simulink model "IDVDSGRA_StatObs_Close"  (R2017b)
settings: Solver=ode4  StartTime=0.0  StopTime=tsim  FixedStep=baseRate  RelTol=1e-3  EnableMultiTasking=on
values from neighbouring files (symbols this model uses):
  baseRate = 0.05    [Run_Initializer.m]
  dockDist = 0.5    [Run_Initializer.m]
  drop_states_BLACK = [ 1.19; 1.45; -0.06737]    [Run_Initializer.m]
  drop_states_RED = [ 2.114; 1.46; -3.113]    [Run_Initializer.m]
  F_thrusters_BLACK = 0.25.*ones(8,1)    [Run_Initializer.m]
  F_thrusters_RED = 0.25.*ones(8,1)    [Run_Initializer.m]
  final_states_BLACK = [1; 0.5; (0/180*pi)]    [Run_Initializer.m]
  fixed_att = init_states_RED(3)    [Run_Initializer.m]
  guess = [8.968203153403679e+02,-2.543974115068790e+03,0.235869606391541,0.474952865321742,0.474987768379695,0.520000000000000,0.485664087948638,0,0,.1,.1,.1,.1,.1,.1,.1,.1,.1,.1,.1,.1,.1,.1,.1,.1,.1,.2]    [Run_Initializer.m]
  home_states_BLACK = [ xLength/2; yLength/2; 0]    [Run_Initializer.m]
  home_states_RED = [ xLength/2+0.4; yLength/2; pi]    [Run_Initializer.m]
  init_states_BLACK = [0.5; 0.5; (0/180*pi)]    [Run_Initializer.m]
  init_states_RED = [ 3; 2; 0]    [Run_Initializer.m]
  Kd_tb = 0.4    [Run_Initializer.m]
  Kd_tr = 0.4    [Run_Initializer.m]
  Kd_xb = 5    [Run_Initializer.m]
  Kd_xr = 5    [Run_Initializer.m]
  Kd_yb = 5    [Run_Initializer.m]
  Kd_yr = 5    [Run_Initializer.m]
  Kp_tb = 0.1    [Run_Initializer.m]
  Kp_tr = 0.1    [Run_Initializer.m]
  Kp_xb = 2    [Run_Initializer.m]
  Kp_xr = 2    [Run_Initializer.m]
  Kp_yb = 2    [Run_Initializer.m]
  Kp_yr = 2    [Run_Initializer.m]
  max_force = F_thrusters_RED(1)*2 * 0.95    [Run_Initializer.m]
  max_torque = 0.13*4    (= 0.52)    [Run_Initializer.m]
  moving_BLACK = [(final_states_BLACK(1)-init_states_BLACK(1))/Phase3_SubPhase2_Duration,(final_states_BLACK(2)-init_states_BLACK(2))/Phase3_SubPhase2_Duration,0]    [Run_Initializer.m]
  noise_variance_BLACK = 0    [Run_Initializer.m]
  noise_variance_RED = 0    [Run_Initializer.m]
  Phase0_End = Phase0_Duration    (= 10)    [Run_Initializer.m]
  Phase1_End = Phase0_Duration + Phase1_Duration    (= 15)    [Run_Initializer.m]
  Phase2_End = Phase0_Duration + Phase1_Duration +                                   Phase2_Duration    (= 35)    [Run_Initializer.m]
  Phase3_Duration = 85    [Run_Initializer.m]
  Phase3_End = Phase0_Duration + Phase1_Duration +                                   Phase2_Duration + Phase3_Duration    (= 120)    [Run_Initializer.m]
  Phase3_SubPhase1_End = Phase2_End + Phase3_SubPhase1_Duration    (= 40)    [Run_Initializer.m]
  Phase3_SubPhase2_Duration = 70    [Run_Initializer.m]
  Phase3_SubPhase2_End = Phase2_End + Phase3_SubPhase1_Duration +                                   Phase3_SubPhase2_Duration    (= 110)    [Run_Initializer.m]
  Phase3_SubPhase3_End = Phase2_End + Phase3_SubPhase1_Duration +                                   Phase3_SubPhase2_Duration +                                  Phase3_SubPhase3_Duration    (= 120)    [Run_Initializer.m]
  Phase3_SubPhase4_End = Phase2_End + Phase3_SubPhase1_Duration +                                   Phase3_SubPhase2_Duration +                                  Phase3_SubPhase3_Duration +                                  Phase3_SubPhase4_Duration    [Run_Initializer.m]
  Phase4_End = Phase0_Duration + Phase1_Duration +                                   Phase2_Duration + Phase3_Duration +                                   Phase4_Duration    (= 140)    [Run_Initializer.m]
  Phase5_End = Phase0_Duration + Phase1_Duration +                                   Phase2_Duration + Phase3_Duration +                                   Phase4_Duration + Phase5_Duration    (= 145)    [Run_Initializer.m]
  REDInertia = 0.2709    [Run_Initializer.m]
  REDMass = 16.9478    [Run_Initializer.m]
  serverRate = 0.1    [Run_Initializer.m]
  thruster_dist2CG_BLACK = [83.42;-52.58;55.94;-60.05;54.08;-53.92;77.06;-55.94]    [Run_Initializer.m]
  thruster_dist2CG_RED = [49.92;-78.08;70.46;-63.54;81.08;-50.42;57.44;-75.96]    [Run_Initializer.m]
  tolSGRA = [Er; Eg]    [Run_Initializer.m]
  xLength = 3.51155    [Run_Initializer.m]
  yLength = 2.41935    [Run_Initializer.m]
undefined symbols (not defined in the file or in its folder): DiscIntNeverNeededParam, platformSelection, simMode
libraries: MainLibrary x22, GPIOLibrary x20, raspberrypilib x17, embdlinuxlib x6, dspsigops x5, dspswit3 x2, simulink x1
(part 8 of 8)

== matlab function IDVDSGRA_StatObs_Close/Phase #5: Hold Home/Change BLACK Behavior/Hough Control/MATLAB Function3 ==
  data: z input; Ox output
function Ox    = C3( z )
%C3 gives the rotation matrix about the z-axis for an angle 'z'
%   z - the angle about the z-axis which you rotate
%   A - the rotation matrix

Ox = [cos(z) sin(z); -sin(z) cos(z)]*[1;0];
end

== matlab function IDVDSGRA_StatObs_Close/Phase #5: Hold Home/Change BLACK Behavior/Hough Control/MATLAB Function4 ==
  data: Oy input; e_out output; e_in input
function e_out = fcn(Oy, e_in)

a = sign(Oy'*e_in);
e_out = -a*norm(e_in);

== matlab function IDVDSGRA_StatObs_Close/Calculate RED_Rz_Shoulder/Wrap2Pi ==
  data: angle_rad input; angle_rad_wrapped output
function angle_rad_wrapped = wrap2pi(angle_rad)

angle_rad_wrapped = angle_rad - 2*pi*floor( (angle_rad+pi)/(2*pi) ); 

end

== matlab function IDVDSGRA_StatObs_Close/Calculate RED_Rz_Elbow/Wrap to [-pi pi] ==
  data: angle_rad input; angle_rad_wrapped output
function angle_rad_wrapped = wrap2pi(angle_rad)

angle_rad_wrapped = angle_rad - 2*pi*floor( (angle_rad+pi)/(2*pi) ); 

end

== matlab function IDVDSGRA_StatObs_Close/Phase #5: Hold Home/Change RED Behavior/Hough Control/MATLAB Function2 ==
  data: Oy output; z input; Ox output
function [Oy, Ox]   = C3( z )
%C3 gives the rotation matrix about the z-axis for an angle 'z'
%   z - the angle about the z-axis which you rotate
%   A - the rotation matrix

Ox = [cos(z) sin(z); -sin(z) cos(z)]*[1;0];
Oy = [cos(z) sin(z); -sin(z) cos(z)]*[0;1];
end

== matlab function IDVDSGRA_StatObs_Close/Phase #5: Hold Home/Change RED Behavior/Hough Control/MATLAB Function3 ==
  data: z input; Ox output
function Ox    = C3( z )
%C3 gives the rotation matrix about the z-axis for an angle 'z'
%   z - the angle about the z-axis which you rotate
%   A - the rotation matrix

Ox = [cos(z) sin(z); -sin(z) cos(z)]*[1;0];
end

== matlab function IDVDSGRA_StatObs_Close/Phase #5: Hold Home/Change RED Behavior/Hough Control/MATLAB Function4 ==
  data: Oy input; e_out output; e_in input
function e_out = fcn(Oy, e_in)

a = sign(Oy'*e_in);
e_out = -a*norm(e_in);

== matlab function IDVDSGRA_StatObs_Close/Calculate RED_Rz_Wrist/Wrap2Pi ==
  data: angle_rad input; angle_rad_wrapped output
function angle_rad_wrapped = wrap2pi(angle_rad)

angle_rad_wrapped = angle_rad - 2*pi*floor( (angle_rad+pi)/(2*pi) ); 

end

== matlab function IDVDSGRA_StatObs_Close/Phase #3: Experiment/Change BLACK Behavior/Sub-Phase #2 /BLACK_Vx2/Wrap1/MATLAB Function ==
  data: u input; wrappedAngle output
function wrappedAngle = wrapAngle(u)

wrappedAngle = atan2(sin(u),cos(u));

end

== matlab function IDVDSGRA_StatObs_Close/Phase #3: Experiment/Change BLACK Behavior/Sub-Phase #2 /BLACK_Vx1/MATLAB Function1 ==
  data: t input; x output; init_Py input; desired_Vy input
function x = fcn(t, init_Py, desired_Vy)

x = init_Py + (desired_Vy * t);

end

== matlab function IDVDSGRA_StatObs_Close/Phase #3: Experiment/Change BLACK Behavior/Sub-Phase #2 /BLACK_Vx/MATLAB Function1 ==
  data: t input; x output; init_Px input; desired_Vx input
function x = fcn(t, init_Px, desired_Vx)

x = init_Px + (desired_Vx * t);

end
